simulink model "battery_pack2_1"  (R2019a)
settings: Solver=VariableStepAuto  StartTime=0.0  StopTime=10  RelTol=1e-3
undefined symbols (not defined in the file): Ion, Lithium
libraries: powerlib x12, electricdrivelib x8
settings Model: SimulationMode=rapid-accelerator  Creator=Shiva Kumar  LastModifiedBy=Shiva Kumar

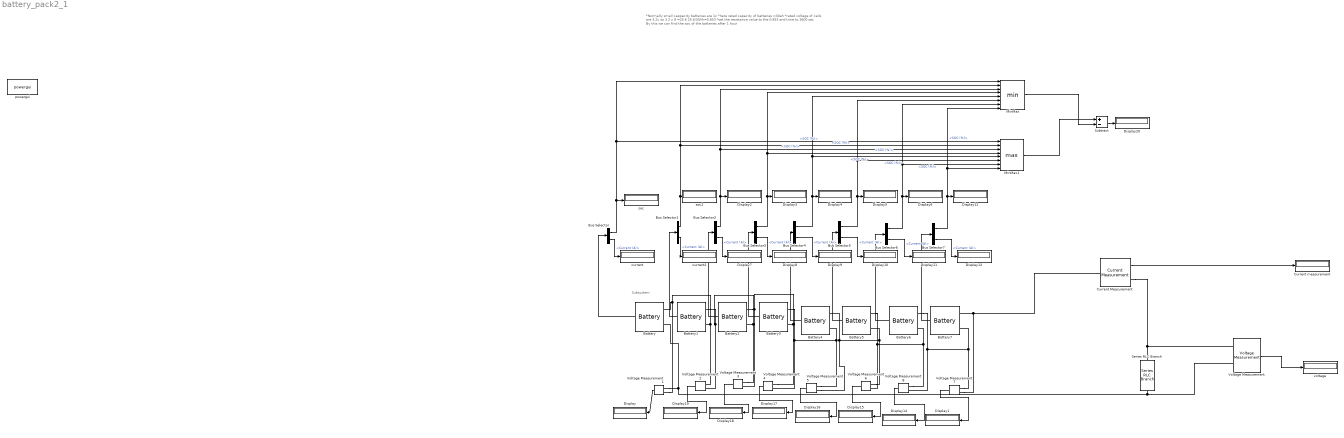
== system battery_pack2_1 ==
  note: *Normally small cappacity batteries are 1c
      | *here rated capacity of batteries =30ah
      | *rated voltage of cells are 3.2v so 3.2 x 8 =25.6
      | 25.6/30Ah=0.853
      | *set the resistance value to the 0.853 and time to 3600 sec
      | By this we can find the soc of the batteries after 1 hour
  note: Subsystem
  Battery : electricdrivelib/Extra Sources/Battery  BatType=Lithium-Ion  ShowTempParam=off  ThermalPreset=no  ShowAgeParam=off  NomV=3.2  NomQ=30  SOC=95  Batt_Tr=30  PresetModel=on  MaxQ=30  MinV=2.4  FullV=3.7248  Dis_rate=13.0435  R=0.0010667  Normal_OP=27.1304  expZone="[3.4572      1.4739]"  current=[6.5 13 32.5]  Units=Time  Tci=20  NomT=20  T2=-30  MaxQ2=4.8  FullV2=7.1  Normal_OP2=5.655  expZone2="[6.58           1]"  Rca=0.6  ti=2000  Dp=0  Neq0=0  Tsim=1e6  Ta1=25  Qeol=5.4*0.9  Reol=0.013333*1.2  Char_age=[2.3478, 3]  Dis_age=[2.3478, 10]  N1=1500  N2=10500  N3=1000  N4=1400  Ta2=45  N5=950
      settings: SourceProductName=Simscape Electrical
  Battery1 : electricdrivelib/Extra Sources/Battery  BatType=Lithium-Ion  ShowTempParam=off  ThermalPreset=no  ShowAgeParam=off  NomV=3.2  NomQ=30  SOC=93  Batt_Tr=30  PresetModel=on  MaxQ=30  MinV=2.4  FullV=3.7248  Dis_rate=13.0435  R=0.0010667  Normal_OP=27.1304  expZone="[3.4572      1.4739]"  current=[6.5 13 32.5]  Units=Time  Tci=20  NomT=20  T2=-30  MaxQ2=4.8  FullV2=7.1  Normal_OP2=5.655  expZone2="[6.58           1]"  Rca=0.6  ti=2000  Dp=0  Neq0=0  Tsim=1e6  Ta1=25  Qeol=5.4*0.9  Reol=0.013333*1.2  Char_age=[2.3478, 3]  Dis_age=[2.3478, 10]  N1=1500  N2=10500  N3=1000  N4=1400  Ta2=45  N5=950
      settings: SourceProductName=Simscape Electrical
  Battery2 : electricdrivelib/Extra Sources/Battery  BatType=Lithium-Ion  ShowTempParam=off  ThermalPreset=no  ShowAgeParam=off  NomV=3.2  NomQ=30  SOC=91  Batt_Tr=30  PresetModel=on  MaxQ=30  MinV=2.4  FullV=3.7248  Dis_rate=13.0435  R=0.0010667  Normal_OP=27.1304  expZone="[3.4572      1.4739]"  current=[6.5 13 32.5]  Units=Time  Tci=20  NomT=20  T2=-30  MaxQ2=4.8  FullV2=7.1  Normal_OP2=5.655  expZone2="[6.58           1]"  Rca=0.6  ti=2000  Dp=0  Neq0=0  Tsim=1e6  Ta1=25  Qeol=5.4*0.9  Reol=0.013333*1.2  Char_age=[2.3478, 3]  Dis_age=[2.3478, 10]  N1=1500  N2=10500  N3=1000  N4=1400  Ta2=45  N5=950
      settings: SourceProductName=Simscape Electrical
  Battery3 : electricdrivelib/Extra Sources/Battery  BatType=Lithium-Ion  ShowTempParam=off  ThermalPreset=no  ShowAgeParam=off  NomV=3.2  NomQ=30  SOC=85  Batt_Tr=30  PresetModel=on  MaxQ=30  MinV=2.4  FullV=3.7248  Dis_rate=13.0435  R=0.0010667  Normal_OP=27.1304  expZone="[3.4572      1.4739]"  current=[6.5 13 32.5]  Units=Time  Tci=20  NomT=20  T2=-30  MaxQ2=4.8  FullV2=7.1  Normal_OP2=5.655  expZone2="[6.58           1]"  Rca=0.6  ti=2000  Dp=0  Neq0=0  Tsim=1e6  Ta1=25  Qeol=5.4*0.9  Reol=0.013333*1.2  Char_age=[2.3478, 3]  Dis_age=[2.3478, 10]  N1=1500  N2=10500  N3=1000  N4=1400  Ta2=45  N5=950
      settings: SourceProductName=Simscape Electrical
  Battery4 : electricdrivelib/Extra Sources/Battery  BatType=Lithium-Ion  ShowTempParam=off  ThermalPreset=no  ShowAgeParam=off  NomV=3.2  NomQ=30  SOC=92  Batt_Tr=30  PresetModel=on  MaxQ=30  MinV=2.4  FullV=3.7248  Dis_rate=13.0435  R=0.0010667  Normal_OP=27.1304  expZone="[3.4572      1.4739]"  current=[6.5 13 32.5]  Units=Time  Tci=20  NomT=20  T2=-30  MaxQ2=4.8  FullV2=7.1  Normal_OP2=5.655  expZone2="[6.58           1]"  Rca=0.6  ti=2000  Dp=0  Neq0=0  Tsim=1e6  Ta1=25  Qeol=5.4*0.9  Reol=0.013333*1.2  Char_age=[2.3478, 3]  Dis_age=[2.3478, 10]  N1=1500  N2=10500  N3=1000  N4=1400  Ta2=45  N5=950
      settings: SourceProductName=Simscape Electrical
  Battery5 : electricdrivelib/Extra Sources/Battery  BatType=Lithium-Ion  ShowTempParam=off  ThermalPreset=no  ShowAgeParam=off  NomV=3.2  NomQ=30  SOC=94  Batt_Tr=30  PresetModel=on  MaxQ=30  MinV=2.4  FullV=3.7248  Dis_rate=13.0435  R=0.0010667  Normal_OP=27.1304  expZone="[3.4572      1.4739]"  current=[6.5 13 32.5]  Units=Time  Tci=20  NomT=20  T2=-30  MaxQ2=4.8  FullV2=7.1  Normal_OP2=5.655  expZone2="[6.58           1]"  Rca=0.6  ti=2000  Dp=0  Neq0=0  Tsim=1e6  Ta1=25  Qeol=5.4*0.9  Reol=0.013333*1.2  Char_age=[2.3478, 3]  Dis_age=[2.3478, 10]  N1=1500  N2=10500  N3=1000  N4=1400  Ta2=45  N5=950
      settings: SourceProductName=Simscape Electrical
  Battery6 : electricdrivelib/Extra Sources/Battery  BatType=Lithium-Ion  ShowTempParam=off  ThermalPreset=no  ShowAgeParam=off  NomV=3.2  NomQ=30  SOC=90  Batt_Tr=30  PresetModel=on  MaxQ=30  MinV=2.4  FullV=3.7248  Dis_rate=13.0435  R=0.0010667  Normal_OP=27.1304  expZone="[3.4572      1.4739]"  current=[6.5 13 32.5]  Units=Time  Tci=20  NomT=20  T2=-30  MaxQ2=4.8  FullV2=7.1  Normal_OP2=5.655  expZone2="[6.58           1]"  Rca=0.6  ti=2000  Dp=0  Neq0=0  Tsim=1e6  Ta1=25  Qeol=5.4*0.9  Reol=0.013333*1.2  Char_age=[2.3478, 3]  Dis_age=[2.3478, 10]  N1=1500  N2=10500  N3=1000  N4=1400  Ta2=45  N5=950
      settings: SourceProductName=Simscape Electrical
  Battery7 : electricdrivelib/Extra Sources/Battery  BatType=Lithium-Ion  ShowTempParam=off  ThermalPreset=no  ShowAgeParam=off  NomV=3.2  NomQ=30  SOC=96  Batt_Tr=30  PresetModel=on  MaxQ=30  MinV=2.4  FullV=3.7248  Dis_rate=13.0435  R=0.0010667  Normal_OP=27.1304  expZone="[3.4572      1.4739]"  current=[6.5 13 32.5]  Units=Time  Tci=20  NomT=20  T2=-30  MaxQ2=4.8  FullV2=7.1  Normal_OP2=5.655  expZone2="[6.58           1]"  Rca=0.6  ti=2000  Dp=0  Neq0=0  Tsim=1e6  Ta1=25  Qeol=5.4*0.9  Reol=0.013333*1.2  Char_age=[2.3478, 3]  Dis_age=[2.3478, 10]  N1=1500  N2=10500  N3=1000  N4=1400  Ta2=45  N5=950
      settings: SourceProductName=Simscape Electrical
  Bus Selector{,1..7} (8 alike) : BusSelector  OutputSignals=SOC (%),Current (A)
  Current Measurement : powerlib/Measurements/Current Measurement  PhasorSimulation=off  OutputType=Complex  PSBequivalent=0
      settings: SourceProductName=Simscape Electrical
  Current measurement : Display
  Display{,1..20} (21 alike) : Display
  MinMax : MinMax  Inputs=8
  MinMax1 : MinMax  Function=max  Inputs=8
  Series RLC Branch : powerlib/Elements/Series RLC Branch  LConnTagsString=__new0  RConnTagsString=__new0  BranchType=R  Resistance=1.5  Inductance=1e-3  SetiL0=off  InitialCurrent=0  Capacitance=1e-6  Setx0=off  InitialVoltage=0  Measurements=None
      settings: SourceProductName=Simscape Electrical
  Subtract : Sum  Inputs=+-
  Voltage Measurement{,1..8} (9 alike) : powerlib/Measurements/Voltage Measurement  PhasorSimulation=off  OutputType=Complex  PSBequivalent=0
      settings: SourceProductName=Simscape Electrical
  current : Display
  current2 : Display
  powergui : powerlib/powergui  Priority=1  SimulationMode=Continuous  SampleTime=50e-6  frequency=60  Iterations=50  frequencyindice=0  Pbase=100e6  ErrMax=1e-4  UnitsV=kV  UnitsW=MW  buscounter=0  FunctionMessages=off  echomessages=off  EnableUseOfTLC=off  CurrentSourceSwitches=off  DisableSnubberDevices=off  DisableRonSwitches=off  DisableVfSwitches=off  DisplayEquations=off  AutomaticDiscreteSolvers=off  SolverType=Tustin/Backward Euler (TBE)  Interpol=off  ExternalGateDelay=off  methode=off  Ts=100  x0status=blocks  SPID=on  SwTol=0  HookPort=off  NonlinearTolerance=0  nMaxIteration=15  ContinueOnMaxIteration=off  RestoreLinks=warning  ResistiveCurrentMeasurement=off  Frange=[0:2:500]  Ylog=off  Xlog=on  ShowGrid=off  save=off  variable=ZData  structure=0  ZoomFFT=off  StartTime=0.0  cycles=1  DisplayStyle=1  fundamental=60  FreqAxis=off  MaxFrequency=1000  frequencyindicesteady=1  RmsSteady=1  display=off
      settings: SourceProductName=Simscape Electrical
  "soc " : Display
  soc2 : Display
  "voltage " : Display
  wires:
  Bus Selector/1 -> MinMax1/1, MinMax/1, "soc "/1  "<SOC (%)>"
  Bus Selector/2 -> current/1  "<Current (A)>"
  Current Measurement/1 -> Current measurement/1
  Voltage Measurement/1 -> "voltage "/1
  Battery/1 -> Bus Selector/1
  Battery1/1 -> Bus Selector1/1
  Battery2/1 -> Bus Selector2/1
  Battery3/1 -> Bus Selector3/1
  Battery4/1 -> Bus Selector4/1
  Battery5/1 -> Bus Selector5/1
  Battery6/1 -> Bus Selector6/1
  Battery7/1 -> Bus Selector7/1
  Bus Selector1/1 -> MinMax1/2, MinMax/2, soc2/1  "<SOC (%)>"
  Bus Selector1/2 -> current2/1  "<Current (A)>"
  Bus Selector2/1 -> MinMax1/3, MinMax/3, Display2/1  "<SOC (%)>"
  Bus Selector2/2 -> Display7/1  "<Current (A)>"
  Bus Selector3/1 -> MinMax1/4, MinMax/4, Display3/1  "<SOC (%)>"
  Bus Selector3/2 -> Display8/1  "<Current (A)>"
  Bus Selector4/1 -> MinMax1/5, MinMax/5, Display4/1  "<SOC (%)>"
  Bus Selector4/2 -> Display9/1  "<Current (A)>"
  Bus Selector5/1 -> MinMax1/6, MinMax/6, Display5/1  "<SOC (%)>"
  Bus Selector5/2 -> Display10/1  "<Current (A)>"
  Bus Selector6/1 -> MinMax1/7, MinMax/7, Display6/1  "<SOC (%)>"
  Bus Selector6/2 -> Display11/1  "<Current (A)>"
  Bus Selector7/1 -> MinMax1/8, MinMax/8, Display12/1  "<SOC (%)>"
  Bus Selector7/2 -> Display13/1  "<Current (A)>"
  Voltage Measurement1/1 -> Display/1
  Voltage Measurement2/1 -> Display19/1
  Voltage Measurement3/1 -> Display18/1
  Voltage Measurement4/1 -> Display17/1
  Voltage Measurement5/1 -> Display16/1
  Voltage Measurement6/1 -> Display15/1
  Voltage Measurement8/1 -> Display14/1
  Voltage Measurement7/1 -> Display1/1
  Subtract/1 -> Display20/1
  MinMax1/1 -> Subtract/1
  MinMax/1 -> Subtract/2
  connections:
  Series RLC Branch/LConn1 -- Current Measurement/RConn1 -- Voltage Measurement/LConn1
  Battery2/LConn1 -- Voltage Measurement3/LConn1 -- Voltage Measurement4/LConn2 -- Battery3/LConn2
  Battery1/LConn1 -- Voltage Measurement3/LConn2 -- Battery2/LConn2 -- Voltage Measurement2/LConn1
  Battery6/LConn1 -- Battery7/LConn2 -- Voltage Measurement7/LConn2 -- Voltage Measurement8/LConn1
  Current Measurement/LConn1 -- Voltage Measurement7/LConn1 -- Battery7/LConn1
  Series RLC Branch/RConn1 -- Battery/LConn2 -- Voltage Measurement1/LConn2 -- Voltage Measurement/LConn2
  Voltage Measurement1/LConn1 -- Battery/LConn1 -- Battery1/LConn2 -- Voltage Measurement2/LConn2
  Battery5/LConn1 -- Battery6/LConn2 -- Voltage Measurement8/LConn2 -- Voltage Measurement6/LConn1
  Voltage Measurement5/LConn1 -- Battery5/LConn2 -- Voltage Measurement6/LConn2 -- Battery4/LConn1
  Battery3/LConn1 -- Battery4/LConn2 -- Voltage Measurement5/LConn2 -- Voltage Measurement4/LConn1
